simulink model "sine_wave_inverter"  (R2020a)
settings: Solver=VariableStepAuto  StartTime=0.0  StopTime=10.0  RelTol=1e-3
libraries: eePwmGenerator x2
settings Model: Creator=kishan  LastModifiedBy=kishan

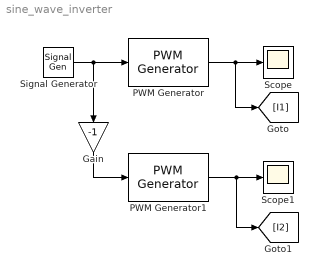
== system sine_wave_inverter ==
  Gain : Gain  Gain=-1
  PWM Generator : eePwmGenerator/PWM Generator  CarrCount=Up  Tper=0.001  Ts=5e-5
  PWM Generator1 : eePwmGenerator/PWM Generator  CarrCount=Up  Tper=0.001  Ts=5e-5
  Scope : Scope
  Scope1 : Scope
  Signal Generator : SignalGenerator  Amplitude=5  Frequency=50
  wires:
  Signal Generator/1 -> Gain/1, PWM Generator/1
  PWM Generator/1 -> [I1], Scope/1
  PWM Generator1/1 -> [I2], Scope1/1
  Gain/1 -> PWM Generator1/1
